simulink model "RBNN_NNT_timing_of_learning_1layerRBNN_openloop1"  (R2019a)
settings: Solver=FixedStepAuto  StartTime=0.0  StopTime=inf  FixedStep=0.000001  RelTol=1e-3
libraries: dspstat3 x6, dspxfrm3 x1
(part 1 of 3)
settings Model: NumberOfSteps=160000  Creator=vardhah  LastModifiedBy=vardhah
settings DataIOCC: ReturnWorkspaceOutputs=off
settings DebuggingCC: UnderSpecifiedDimensionMsg=warning  ArithmeticOperatorsInVariantConditions=warning

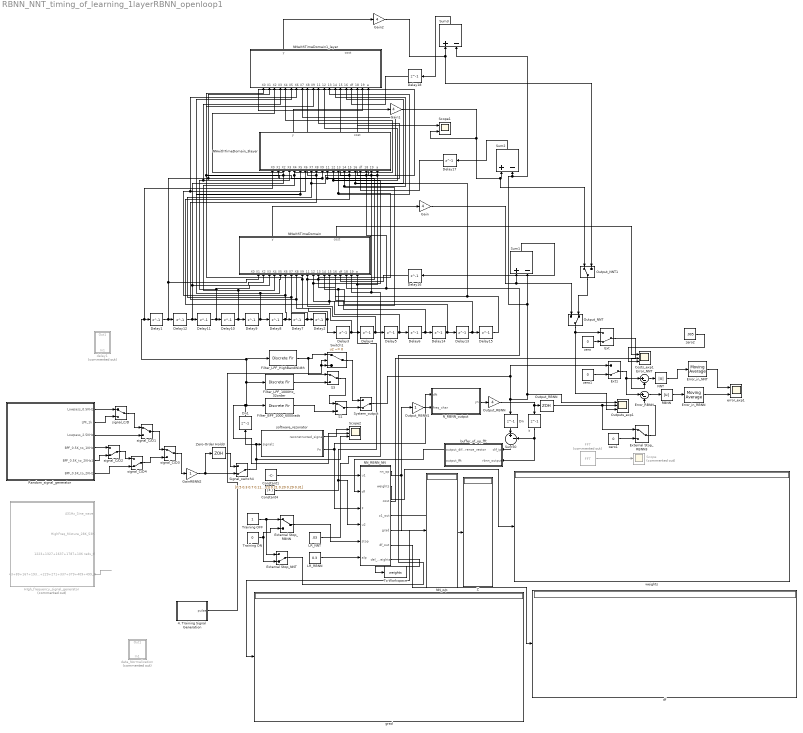
== system RBNN_NNT_timing_of_learning_1layerRBNN_openloop1 ==
  4. Training Signal Generation : MATLAB Function  TreatAsAtomicUnit=on
  Constant1 : Constant  Value=[0.5 0.3 0.7 0.11 0.13 0.19 0.2 0.9 0.8 0.17 0.19 0.23 0.21 0.20 0.29 0.31]
  Constant4 : Constant  Value=[3 ]
  Costs_exp1 : Scope  NumInputPorts=3
  Delay{1..18} (18 alike) : Delay  DelayLength=1  InitialCondition=0
  Dn : Delay  DelayLength=1  InitialCondition=0
  Dn1 : Delay  DelayLength=1  InitialCondition=0
  Error_NNT : Sum  Inputs=|+-
  Error_RBNN : Sum  Inputs=|+-
  Error_in_NNT : dspstat3/Moving Average  Method=Sliding window  ForgettingFactorPort=off  SpecifyWindowLength=on  WindowLength=32  ForgettingFactor=0.9  SimulateUsing=Code generation
  Error_in_RBNN : dspstat3/Moving Average  Method=Sliding window  ForgettingFactorPort=off  SpecifyWindowLength=on  WindowLength=32  ForgettingFactor=0.9  SimulateUsing=Code generation
  Ext : ManualSwitch  CurrentSetting=0
  Ext1 : ManualSwitch  CurrentSetting=0
  External Stop_NNT : ManualSwitch  CurrentSetting=0
  External Stop_RBNN : ManualSwitch
  External Stop_RBNN3 : ManualSwitch
  FFT : dspxfrm3/FFT  Commented=on  FFTImplementation=Auto  CompMethod=Table lookup  TableOpt=NEW  TableOptActive=Speed  BitRevOrder=off  Normalize=off  InheritFFTLength=off  FFTLength=16  WrapInput=on  roundingMode=Floor  overflowMode=off  firstCoeffDataTypeStr=Inherit: Same word length as input  firstCoeffLastDataTypeStr=Inherit: Same word length as input  outputMin=[]  outputMax=[]
  Filter_BPF_1000_6000rads : DiscreteFir  Tag=BlockMethodSubSystem  Coefficients=[-0.00618210440285905504 -0.0303096045628865642 -0.0409410179735487934 -0.0229077272949628416 -0.00102866067847521788 -0.0105080795115171741 -0.046522204158505033 -0.0628979042424121088 -0.0316879488224668174 0.0100728634546924985 -0.00266882733070159146 -0.0740228240448953662 -0.116856903059740558 -0.0367740036181566435 0.151619332309241961 0.312853708085660598 0.312853708085660598 0.151619332309241961 -0.0367740036181566435 -0.116856903059740558 -0.0740228240448953662 -0.00266882733070159146 0.0100728634546924985 -0.0316879488224668174 -0.0628979042424121088 -0.046522204158505033 -0.0105080795115171741 -0.00102866067847521788 -0.0229077272949628416 -0.0409410179735487934 -0.0303096045628865642 -0.00618210440285905504]  InputProcessing=Columns as channels (frame based)  SampleTime=0.0001
  Filter_LPF_1000Hz_32order : DiscreteFir  Tag=BlockMethodSubSystem  Coefficients=[-0.0630584015316483504 0.00280766392327516656 0.0141040221857817727 0.0270919956895751823 0.0349204038453045582 0.0318455482714793056 0.016337666727450996 -0.00752756764241900578 -0.0304914391413993666 -0.0410993624858043 -0.0297930254792096449 0.0068075382499173942 0.0640229913309069559 0.129444538808950849 0.186430196276218318 0.21962321117281583 0.21962321117281583 0.186430196276218318 0.129444538808950849 0.0640229913309069559 0.0068075382499173942 -0.0297930254792096449 -0.0410993624858043 -0.0304914391413993666 -0.00752756764241900578 0.016337666727450996 0.0318455482714793056 0.0349204038453045582 0.0270919956895751823 0.0141040221857817727 0.00280766392327516656 -0.0630584015316483504]  InputProcessing=Columns as channels (frame based)  SampleTime=0.0001
  Filter_LPF_HighBandWidth : DiscreteFir  Tag=BlockMethodSubSystem  Coefficients=[0.00257561197553052117 0.0149226993015543988 -0.0126813197622564593 0.0131583623867790739 -0.0109438145213804211 0.00462377218068549256 0.00574880781840408916 -0.0188595701191665473 0.032156879848246514 -0.042054633169390801 0.0443249918452583783 -0.0343435917303160365 0.00670297923827019304 0.0478068572768818173 -0.160206703181909604 0.618531838092966302 0.618531838092966302 -0.160206703181909604 0.0478068572768818173 0.00670297923827019304 -0.0343435917303160365 0.0443249918452583783 -0.042054633169390801 0.032156879848246514 -0.0188595701191665473 0.00574880781840408916 0.00462377218068549256 -0.0109438145213804211 0.0131583623867790739 -0.0126813197622564593 0.0149226993015543988 0.00257561197553052117]  InputProcessing=Columns as channels (frame based)  SampleTime=0.0001
  Gain : Gain  Gain=4
  Gain1 : Gain  Gain=4
  Gain2 : Gain  Gain=4
  GainRBNN2 : Gain
  HIgh_frequency_signal_generator : Subsystem  Commented=on
  LR_NNT : Constant  Value=.03
  LR_RBNN : Constant  Value=0.3
  NNT : Abs
  NN_RBNN_NN : MATLAB Function  TreatAsAtomicUnit=on
  NN_o/p : Display
  NNwithTimeDomain : MATLAB Function  TreatAsAtomicUnit=on  SystemSampleTime=0.0001
  NNwithTimeDomain1_layer : MATLAB Function  TreatAsAtomicUnit=on  SystemSampleTime=0.0001
  NNwithTimeDomain_3layer : MATLAB Function  TreatAsAtomicUnit=on  SystemSampleTime=0.0001
  N_RBNN_output : MATLAB Function  TreatAsAtomicUnit=on
  Output_NNT : ManualSwitch  CurrentSetting=0
  Output_NNT1 : ManualSwitch
  Output_RBNN : Gain  Gain=4
  "Output_RBNN " : ZeroOrderHold  SampleTime=-1
  Output_RBNN1 : Gain
  Outputs_exp1 : Scope  NumInputPorts=3
  RBNN : Abs
  Random_signal_generator : Subsystem
  S1 : ManualSwitch
  S3 : ManualSwitch
  Scope : Scope  Commented=on
  Scope1 : Scope  NumInputPorts=2
  Scope2 : Scope  NumInputPorts=3
  Signal_switch4 : ManualSwitch  CurrentSetting=0
  Sum1 : Sum  Inputs=+-
  Sum2 : Sum  Inputs=+-
  Sum3 : Sum  Inputs=+-
  Sum50 : Sum  Inputs=|+-
  Switch1 : Switch  Criteria=u2 ~= 0
  "System_output " : ManualSwitch  CurrentSetting=0
  To Workspace : ToWorkspace  VariableName=weights  SaveFormat=Timeseries  SampleTime=-1
  Training OFF : Constant
  Training ON : Constant  Value=0
  Z : Display
  Zero-Order Hold3 : ZeroOrderHold  SampleTime=0.0001
  buffer_of_op_fft : MATLAB Function  TreatAsAtomicUnit=on
  data_Normalization : Subsystem  Commented=on
  delay1 : Subsystem  Commented=on
  df : Display
  error_exp1 : Scope  NumInputPorts=2
  grad : Display
  signal_C/D : ManualSwitch
  signal_C/D1 : ManualSwitch
  signal_C/D2 : ManualSwitch  CurrentSetting=0
  signal_C/D3 : ManualSwitch
  signal_C/D4 : ManualSwitch  CurrentSetting=0
  software_rezonator : MATLAB Function  TreatAsAtomicUnit=on  SystemSampleTime=0.0001
  weights : Display
  y : Delay  DelayLength=1  InitialCondition=0
  zero : Constant  Value=0
  zero1 : Constant  Value=0
  "zero1 " : Constant  Value=0
  zero2 : Constant  Value=.005
  wires:
  software_rezonator/1(reconstructed_signal) -> Scope2/1
  software_rezonator/2(Fn) -> NN_RBNN_NN/3(F), N_RBNN_output/1(dft)
  N_RBNN_output/1(yn) -> Output_RBNN/1
  Dn/1 -> Sum50/1
  y/1 -> buffer_of_op_fft/2(rbnn_output), Sum50/2
  NN_RBNN_NN/1(nn_op) -> NN_o/p/1, Output_RBNN1/1
  Training OFF/1 -> External Stop_NNT/1, External Stop_RBNN/1
  Training ON/1 -> External Stop_NNT/2, External Stop_RBNN/2
  NN_RBNN_NN/3(cost) -> Costs_exp1/2
  NN_RBNN_NN/2(weights) -> weights/1
  NN_RBNN_NN/4(z1_out) -> Z/1
  Sum50/1 -> buffer_of_op_fft/1(dif_ip)
  NNwithTimeDomain/1(y) -> Gain/1
  Delay16/1 -> NNwithTimeDomain/17(df)
  Delay4/1 -> NNwithTimeDomain_3layer/11(X10), NNwithTimeDomain1_layer/11(X10), NNwithTimeDomain/11(X10), Delay5/1
  Delay6/1 -> Delay14/1, NNwithTimeDomain_3layer/13(X12), NNwithTimeDomain1_layer/13(X12), NNwithTimeDomain/13(X12)
  Delay5/1 -> NNwithTimeDomain_3layer/12(X11), NNwithTimeDomain1_layer/12(X11), NNwithTimeDomain/12(X11), Delay6/1
  NNwithTimeDomain/2(cost) -> Costs_exp1/1
  Delay2/1 -> Delay3/1, NNwithTimeDomain1_layer/9(X8), NNwithTimeDomain_3layer/9(X8), NNwithTimeDomain/9(X8)
  Delay15/1 -> NNwithTimeDomain_3layer/16(X15), NNwithTimeDomain1_layer/16(X15), NNwithTimeDomain/16(X15)
  Delay13/1 -> NNwithTimeDomain/15(X14), NNwithTimeDomain1_layer/15(X14), NNwithTimeDomain_3layer/15(X14), Delay15/1
  Delay14/1 -> NNwithTimeDomain_3layer/14(X13), NNwithTimeDomain1_layer/14(X13), NNwithTimeDomain/14(X13), Delay13/1
  Delay10/1 -> NNwithTimeDomain/5(X4), NNwithTimeDomain1_layer/5(X4), NNwithTimeDomain_3layer/5(X4), Delay9/1
  GainRBNN2/1 -> Zero-Order Hold3/1, Signal_switch4/2
  Delay3/1 -> Delay4/1, NNwithTimeDomain1_layer/1(X0), NNwithTimeDomain_3layer/10(X9), NNwithTimeDomain1_layer/10(X9), NNwithTimeDomain/10(X9)
  Delay7/1 -> Delay2/1, NNwithTimeDomain_3layer/8(X7), NNwithTimeDomain1_layer/8(X7), NNwithTimeDomain/8(X7)
  Delay8/1 -> NNwithTimeDomain_3layer/7(X6), NNwithTimeDomain1_layer/7(X6), NNwithTimeDomain/7(X6), Delay7/1
  Delay1/1 -> NNwithTimeDomain1_layer/2(X1), NNwithTimeDomain_3layer/2(X1), NNwithTimeDomain/2(X1), Delay12/1
  Delay9/1 -> Delay8/1, NNwithTimeDomain/6(X5), NNwithTimeDomain_3layer/6(X5), NNwithTimeDomain1_layer/6(X5)
  Delay12/1 -> NNwithTimeDomain1_layer/3(X2), NNwithTimeDomain_3layer/3(X2), NNwithTimeDomain/3(X2), Delay11/1
  Delay11/1 -> Delay10/1, NNwithTimeDomain_3layer/4(X3), NNwithTimeDomain1_layer/4(X3), NNwithTimeDomain/4(X3)
  Sum1/1 -> Delay16/1
  Error_RBNN/1 -> RBNN/1
  Error_NNT/1 -> NNT/1
  Gain/1 -> Output_NNT/1, Sum1/1
  LR_RBNN/1 -> NN_RBNN_NN/6(alp)
  RBNN/1 -> Error_in_RBNN/1
  NNT/1 -> Error_in_NNT/1
  Error_in_NNT/1 -> error_exp1/1
  Error_in_RBNN/1 -> error_exp1/2
  External Stop_NNT/1 -> NNwithTimeDomain1_layer/18(stop), NNwithTimeDomain_3layer/18(stop), NNwithTimeDomain/18(stop)
  Output_RBNN/1 -> y/1, "Output_RBNN "/1
  LR_NNT/1 -> NNwithTimeDomain1_layer/19(alpha_l), NNwithTimeDomain_3layer/19(alpha_l), NNwithTimeDomain/19(alpha_l)
  HIgh_frequency_signal_generator/4(43+89+167+193+229+271+337+379+409+499_H) -> ?
  Zero-Order Hold3/1 -> Signal_switch4/1
  FFT/1 -> Scope/1
  Switch1/1 -> "System_output "/1
  Constant1/1 -> NN_RBNN_NN/1(u1)
  4. Training Signal Generation/1(pulse) -> Switch1/3, Switch1/2
  Constant4/1 -> NNwithTimeDomain1_layer/20(a), NNwithTimeDomain_3layer/20(a), NNwithTimeDomain/20(a), NN_RBNN_NN/4(u2)
  NNwithTimeDomain_3layer/1(y) -> Gain1/1
  Gain1/1 -> Scope1/2, Output_NNT1/1, Sum2/1
  Sum2/1 -> Delay17/1
  Delay17/1 -> NNwithTimeDomain_3layer/17(df)
  NNwithTimeDomain_3layer/2(cost) -> Scope1/1
  Output_NNT/1 -> Outputs_exp1/3, Ext/1
  Filter_LPF_1000Hz_32order/1 -> S3/2
  S3/1 -> S1/1
  Filter_BPF_1000_6000rads/1 -> S1/2
  S1/1 -> "System_output "/2
  Filter_LPF_HighBandWidth/1 -> S3/1, Switch1/1
  Output_RBNN1/1 -> N_RBNN_output/2(freq_char)
  NN_RBNN_NN/5(grad) -> grad/1
  "Output_RBNN "/1 -> External Stop_RBNN3/1, Outputs_exp1/2
  NN_RBNN_NN/6(df_out) -> df/1
  "System_output "/1 -> Ext1/1, Dn/1, Sum3/2, Sum2/2, Sum1/2, Outputs_exp1/1
  NN_RBNN_NN/7(del_weights) -> To Workspace/1
  Signal_switch4/1 -> Scope2/3, Dn1/1, software_rezonator/1(signalz)
  Dn1/1 -> Filter_BPF_1000_6000rads/1, Filter_LPF_1000Hz_32order/1, NNwithTimeDomain_3layer/1(X0), Delay1/1, Filter_LPF_HighBandWidth/1, Scope2/2
  signal_C/D/1 -> signal_C/D1/1
  Random_signal_generator/3(Lowpass_2.5KHz) -> signal_C/D1/2
  Random_signal_generator/4(BPF_0.5K_to_1KHz) -> signal_C/D2/1
  signal_C/D3/1 -> GainRBNN2/1
  signal_C/D1/1 -> signal_C/D3/1
  Random_signal_generator/1(Lowpass_0.5KHz) -> signal_C/D/1
  Random_signal_generator/2(LPF_1k) -> signal_C/D/2
  "zero1 "/1 -> External Stop_RBNN3/2
  External Stop_RBNN3/1 -> Error_RBNN/2
  Ext/1 -> Error_NNT/2
  zero/1 -> Ext/2
  zero1/1 -> Ext1/2
  Ext1/1 -> Error_RBNN/1, Error_NNT/1
  zero2/1 -> Costs_exp1/3
  Random_signal_generator/5(BPF_0.5K_to_2KHz1) -> signal_C/D2/2
  signal_C/D2/1 -> signal_C/D4/1
  Random_signal_generator/6(BPF_0.5K_to_2KHz) -> signal_C/D4/2
  signal_C/D4/1 -> signal_C/D3/2
  Sum3/1 -> Delay18/1
  Delay18/1 -> NNwithTimeDomain1_layer/17(df)
  NNwithTimeDomain1_layer/1(y) -> Gain2/1
  Gain2/1 -> Output_NNT1/2, Sum3/1
  Output_NNT1/1 -> Output_NNT/2
  buffer_of_op_fft/1(output_difference_vector) -> NN_RBNN_NN/2(df)
  External Stop_RBNN/1 -> NN_RBNN_NN/5(stop)

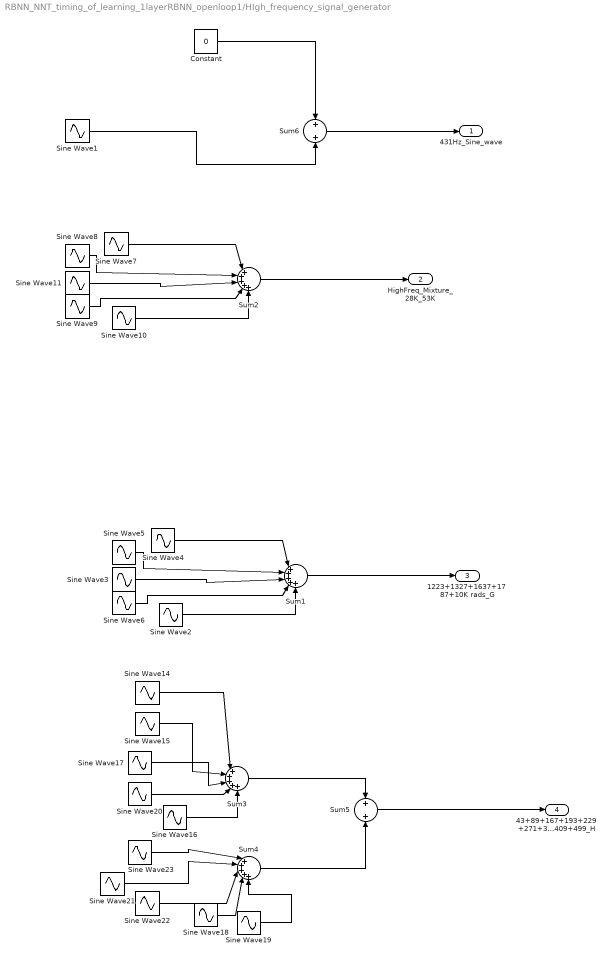
== system RBNN_NNT_timing_of_learning_1layerRBNN_openloop1/HIgh_frequency_signal_generator ==
  Constant : Constant  Value=0
  Sine Wave1 : Sin  Amplitude=0.5  Frequency=23000  SampleTime=0
  Sine Wave10 : Sin  Amplitude=0.5  Frequency=7000  SampleTime=0
  Sine Wave11 : Sin  Amplitude=2  Frequency=3637  SampleTime=0
  Sine Wave14 : Sin  Amplitude=0.1  Frequency=43  SampleTime=0
  Sine Wave15 : Sin  Amplitude=0.1  Frequency=89  SampleTime=0
  Sine Wave16 : Sin  Amplitude=0.1  Frequency=229  SampleTime=0
  Sine Wave17 : Sin  Amplitude=0.1  Frequency=167  SampleTime=0
  Sine Wave18 : Sin  Amplitude=0.1  Frequency=409  SampleTime=0
  Sine Wave19 : Sin  Amplitude=0.1  Frequency=499  SampleTime=0
  Sine Wave2 : Sin  Amplitude=0  Frequency=5000  SampleTime=0
  Sine Wave20 : Sin  Amplitude=0.1  Frequency=193  SampleTime=0
  Sine Wave21 : Sin  Amplitude=0.1  Frequency=337  SampleTime=0
  Sine Wave22 : Sin  Amplitude=0.1  Frequency=379  SampleTime=0
  Sine Wave23 : Sin  Amplitude=0.1  Frequency=271  SampleTime=0
  Sine Wave3 : Sin  Amplitude=0.25  Frequency=200  SampleTime=0
  Sine Wave4 : Sin  Amplitude=0.25  Frequency=50  SampleTime=0
  Sine Wave5 : Sin  Amplitude=0.25  Frequency=100  SampleTime=0
  Sine Wave6 : Sin  Amplitude=0.25  Frequency=1787  SampleTime=0
  Sine Wave7 : Sin  Amplitude=2  Frequency=2230  SampleTime=0
  Sine Wave8 : Sin  Amplitude=2  Frequency=5927  SampleTime=0
  Sine Wave9 : Sin  Amplitude=2  Frequency=3787  SampleTime=0
  Sum{1..4} (4 alike) : Sum  Inputs=|+++++
  Sum5 : Sum
  Sum6 : Sum
  431Hz_Sine_wave : Outport
  HighFreq_Mixture_28K_53K : Outport  Port=2
  1223+1327+1637+1787+10K rads_G : Outport  Port=3
  43+89+167+193+229+271+337+379+409+499_H : Outport  Port=4
  wires:
  Sine Wave9/1 -> Sum2/4
  Sine Wave7/1 -> Sum2/1
  Sine Wave10/1 -> Sum2/5
  Sine Wave8/1 -> Sum2/2
  Sine Wave11/1 -> Sum2/3
  Sum2/1 -> HighFreq_Mixture_28K_53K/1
  Sine Wave23/1 -> Sum4/1
  Sine Wave17/1 -> Sum3/3
  Sine Wave22/1 -> Sum4/3
  Sine Wave18/1 -> Sum4/4
  Sine Wave19/1 -> Sum4/5
  Sine Wave5/1 -> Sum1/2
  Sine Wave20/1 -> Sum3/4
  Sine Wave4/1 -> Sum1/1
  Sine Wave14/1 -> Sum3/1
  Sine Wave15/1 -> Sum3/2
  Sine Wave21/1 -> Sum4/2
  Sine Wave16/1 -> Sum3/5
  Sine Wave6/1 -> Sum1/4
  Sum4/1 -> Sum5/2
  Sum3/1 -> Sum5/1
  Sine Wave2/1 -> Sum1/5
  Sine Wave3/1 -> Sum1/3
  Sum1/1 -> 1223+1327+1637+1787+10K rads_G/1
  Sum5/1 -> 43+89+167+193+229+271+337+379+409+499_H/1
  Sine Wave1/1 -> Sum6/2
  Constant/1 -> Sum6/1
  Sum6/1 -> 431Hz_Sine_wave/1
